simulink model "SampleTime_ejemplo"  (Simulink 7.1)
settings: Solver=ode45  StartTime=0.0  StopTime=10.0  RelTol=1e-3
settings Model: Creator=Usuario  LastModifiedBy=Usuario

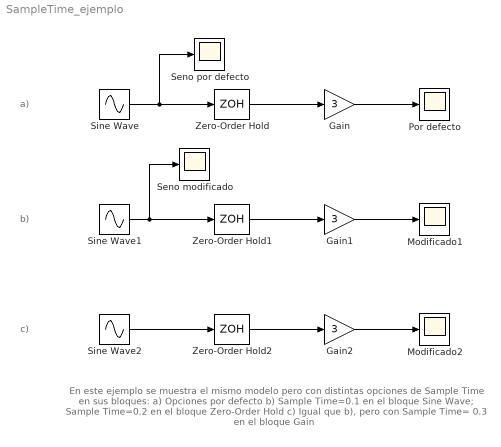
== system SampleTime_ejemplo ==
  note: En este ejemplo se muestra el mismo modelo pero con distintas opciones de Sample Time en sus bloques:
      | a) Opciones por defecto
      | b) Sample Time=0.1 en el bloque Sine Wave; Sample Time=0.2 en el bloque Zero-Order Hold
      | c) Igual que b), pero con Sample Time= 0.3 en el bloque Gain
  note: a)
  note: b)
  note: c)
  Gain : Gain  Gain=3  ParameterDataType=sfix(16)  ParameterScaling=2^0  OutDataType=sfix(16)  OutScaling=2^0
  Gain1 : Gain  Gain=3  ParameterDataType=sfix(16)  ParameterScaling=2^0  OutDataType=sfix(16)  OutScaling=2^0
  Gain2 : Gain  Gain=3  ParameterDataType=sfix(16)  ParameterScaling=2^0  OutDataType=sfix(16)  OutScaling=2^0  SampleTime=0.3
  Modificado1 : Scope
  Modificado2 : Scope
      settings: SaveName=ScopeData4
  Por defecto : Scope
  Seno modificado : Scope
      settings: SaveName=ScopeData3
  Seno por defecto : Scope
      settings: SaveName=ScopeData2
  Sine Wave : Sin  SampleTime=0
  Sine Wave1 : Sin  SampleTime=0.1
  Sine Wave2 : Sin  SampleTime=0.1
  Zero-Order Hold : ZeroOrderHold
  Zero-Order Hold1 : ZeroOrderHold  SampleTime=0.2
  Zero-Order Hold2 : ZeroOrderHold  SampleTime=0.2
  wires:
  Sine Wave/1 -> Zero-Order Hold/1, Seno por defecto/1
  Zero-Order Hold/1 -> Gain/1
  Gain/1 -> Por defecto/1
  Sine Wave1/1 -> Zero-Order Hold1/1, Seno modificado/1
  Zero-Order Hold1/1 -> Gain1/1
  Gain1/1 -> Modificado1/1
  Sine Wave2/1 -> Zero-Order Hold2/1
  Zero-Order Hold2/1 -> Gain2/1
  Gain2/1 -> Modificado2/1
